simulink model "ad_single_dual"  (Simulink 8.9)
settings: Solver=VariableStepAuto  StartTime=0.0  StopTime=10.0  RelTol=1e-3
libraries: MAIv2DAQ x2
settings Model: Creator=Support  LastModifiedBy=torsten
settings DataIOCC: LimitDataPoints=off  SaveFormat=Dataset  SignalLoggingSaveFormat=Dataset
settings OptimizationCC: LifeSpan=auto
settings DebuggingCC: UnderspecifiedInitializationDetection=Simplified  MergeDetectMultiDrivingBlocksExec=error  FcnCallInpInsideContextMsg=error  StateNameClashWarn=none  SFUnexpectedBacktrackingDiag=error  SFNoUnconditionalDefaultTransitionDiag=error  SFExecutionAtInitializationDiag=warning
settings HardwareCC: ProdBitPerPointer=64  ProdBitPerSizeT=64  ProdBitPerPtrDiffT=64  ProdLargestAtomicFloat=Float  ProdIntDivRoundTo=Zero  ProdEndianess=LittleEndian  ProdWordSize=64  ProdHWDeviceType=Intel->x86-64 (Windows64)
settings ModelReferenceCC: PropagateSignalLabelsOutOfModel=on
settings GRTTargetCC: TargetLangStandard=C99 (ISO)  GeneratePreprocessorConditionals=Use local settings  CombineOutputUpdateFcns=on  GRTInterface=off
settings ConfigComp: CovMetricSettings=dwe  CovHtmlReporting=off  CovSaveCumulativeToWorkspaceVar=off  CovSaveSingleToWorkspaceVar=off  CovExternalEMLEnable=on

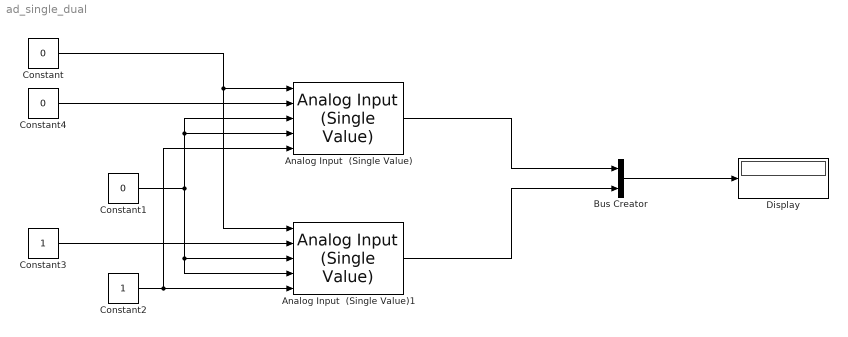
== system ad_single_dual ==
  Analog Input  (Single Value) : MAIv2DAQ/Analog Input/Analog Input  (Single Value)  Device=0  Channel=0  Oversampling=disable  Gain=1
  Analog Input  (Single Value)1 : MAIv2DAQ/Analog Input/Analog Input  (Single Value)  Device=0  Channel=0  Oversampling=disable  Gain=1
  Bus Creator : BusCreator  Inputs=2
  Constant : Constant  Value=0
  Constant1 : Constant  Value=0
  Constant2 : Constant
  Constant3 : Constant
  Constant4 : Constant  Value=0
  Display : Display
      settings: Decimation=2
  wires:
  Analog Input  (Single Value)/1 -> Bus Creator/1
  Analog Input  (Single Value)1/1 -> Bus Creator/2
  Bus Creator/1 -> Display/1
  Constant/1 -> Analog Input  (Single Value)1/1, Analog Input  (Single Value)/1
  Constant1/1 -> Analog Input  (Single Value)1/4, Analog Input  (Single Value)1/3, Analog Input  (Single Value)/4, Analog Input  (Single Value)/3
  Constant2/1 -> Analog Input  (Single Value)1/5, Analog Input  (Single Value)/5
  Constant3/1 -> Analog Input  (Single Value)1/2
  Constant4/1 -> Analog Input  (Single Value)/2
